simulink model "week1problem3"  (R2020b)
settings: Solver=VariableStepAuto  StartTime=0.0  StopTime=10.0  RelTol=1e-3
model workspace (MAT data in the model file):
  k = 0.5792
settings Model: OrderedModelArguments=off  Creator=HP  LastModifiedBy=HP

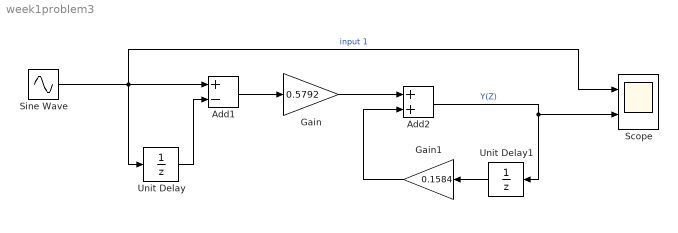
== system week1problem3 ==
  Add1 : Sum  Inputs=+-
  Add2 : Sum
  Gain : Gain  Gain=0.5792
  Gain1 : Gain  Gain=0.1584
  Scope : Scope  NumInputPorts=2
  Sine Wave : Sin  Frequency=300  SampleTime=0
  Unit Delay : UnitDelay  SampleTime=-1  HasFrameUpgradeWarning=on
  Unit Delay1 : UnitDelay  SampleTime=-1  HasFrameUpgradeWarning=on
  wires:
  Gain1/1 -> Add2/2
  Sine Wave/1 -> Scope/1, Add1/1, Unit Delay/1  "input 1"
  Unit Delay/1 -> Add1/2
  Add2/1 -> Scope/2, Unit Delay1/1  "Y(Z)"
  Gain/1 -> Add2/1
  Add1/1 -> Gain/1
  Unit Delay1/1 -> Gain1/1
